simulink model "ex22_simulink"  (R2021b)
settings: Solver=VariableStepAuto  StartTime=0.0  StopTime=50.0  RelTol=1e-3
values from neighbouring files (symbols this model uses):
  D = [ 1,2,4]    [ex10.m]    (also in ex22.m = 0.4; ex23.m = 0.1; ex34.m = [C(2) C(4);d1 0])
  g = 9.8    [ex19.m]    (also in ex22.m)
  j = 1    [ex22.m]
  K = 1    [ex10.m]    (also in ex22.m)
  M = 1    [ex10.m]    (also in ex22.m = 5)
  R = Rv(n)    [ex10.m]    (also in ex22.m = 0.2; ex23.m = 1.3; ex27c.m = 2.8; ex8.m = 10)
settings Model: Creator=rafam  LastModifiedBy=rafam

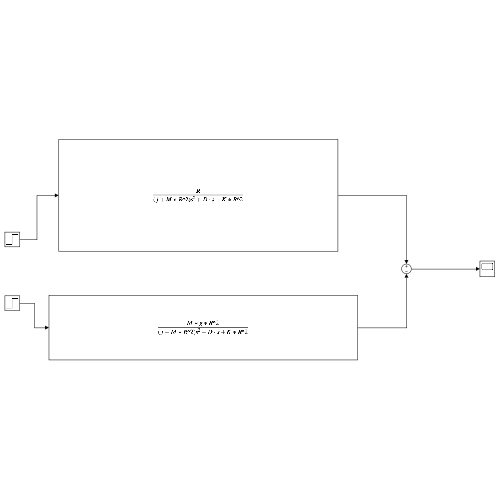
[thumbnail: Simulink's stored preview of the top-level diagram]
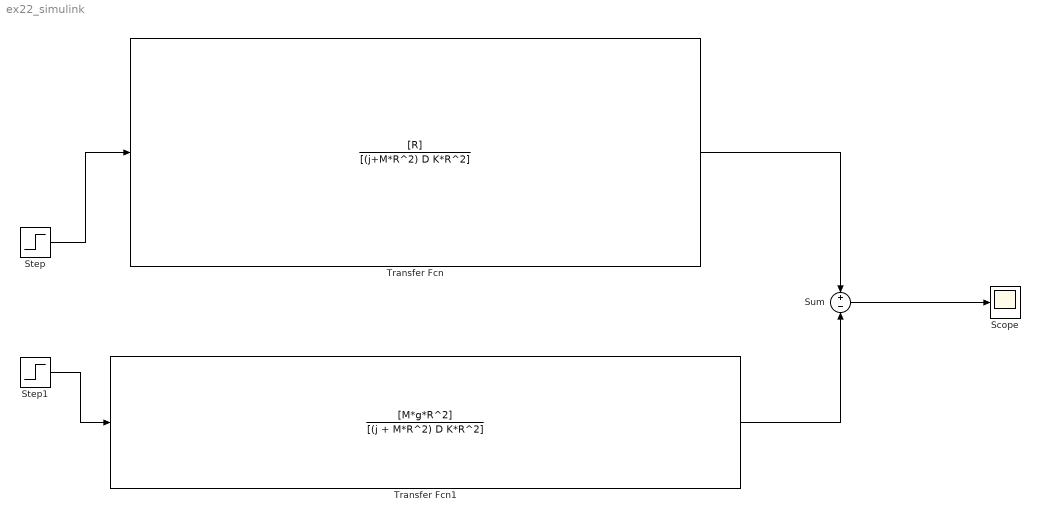
== system ex22_simulink ==
  Scope : Scope
  Step : Step  Time=0  After=10  SampleTime=0
  Step1 : Step  Time=0  SampleTime=0
  Sum : Sum  Inputs=+|-
  Transfer Fcn : TransferFcn  Numerator=[R]  Denominator=[(j+M*R^2) D K*R^2]
  Transfer Fcn1 : TransferFcn  Numerator=[M*g*R^2]  Denominator=[(j + M*R^2) D K*R^2]
  wires:
  Step/1 -> Transfer Fcn/1
  Step1/1 -> Transfer Fcn1/1
  Sum/1 -> Scope/1
  Transfer Fcn/1 -> Sum/1
  Transfer Fcn1/1 -> Sum/2
